simulink model "mov_rot_simulink"  (R2024b)
settings: Solver=VariableStepAuto  StartTime=0.0  StopTime=10.0  MaxStep=0.01  RelTol=1e-3
InitFcn:
  | m = 10;    % kg
  | r = 0.05;  % m
  | k = 100;   % N/m

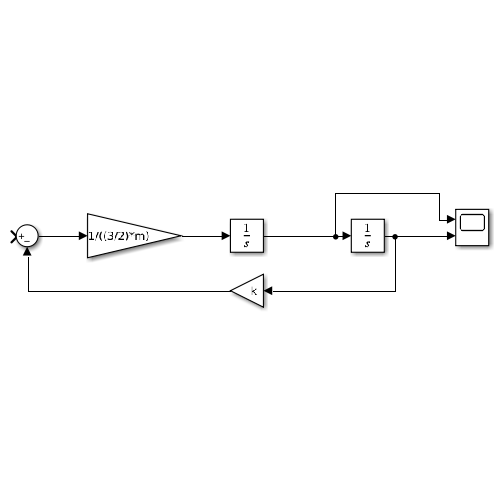
[thumbnail: Simulink's stored preview of the top-level diagram]
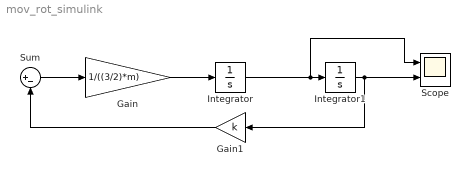
== system mov_rot_simulink ==
  Gain : Gain  Gain=1/((3/2)*m)
  Gain1 : Gain  Gain=k
  Integrator : Integrator  InitialCondition=2
  Integrator1 : Integrator
  Scope : Scope  NumInputPorts=2
  Sum : Sum  Inputs=|+-
  wires:
  Integrator/1 -> Scope/1, Integrator1/1
  Gain/1 -> Integrator/1
  Integrator1/1 -> Gain1/1, Scope/2
  Sum/1 -> Gain/1
  Gain1/1 -> Sum/2
